simulink model "ExRobotAndEnvironmentController"  (Simulink 8.3)
settings: Solver=ode45  StartTime=0.0  StopTime=1000  FixedStep=.01  RelTol=1e-3
undefined symbols (not defined in the file): Env, INITIAL_ROBOT_POS_THETA, INITIAL_ROBOT_POS_X, INITIAL_ROBOT_POS_Y, INTER_WHEEL_DISTANCE, ki_teta, kp_teta, MAX_SPEED, Robot, RobotInit, ts, ts_anim
libraries: simulink x4
settings Model: Creator=alex  LastModifiedBy=schuhm
settings OptimizationCC: ExpressionDepthLimit=2147483647
settings DebuggingCC: SolverPrmCheckMsg=none  FcnCallInpInsideContextMsg=UseLocalSettings
settings SFSimCC: SimParseCustomCode=off

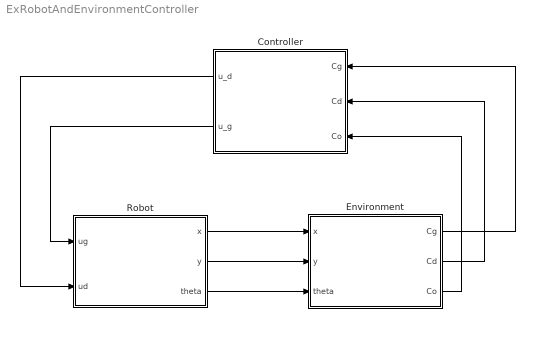
== system ExRobotAndEnvironmentController ==
  Controller : Subsystem
  Environment : Subsystem
  Robot : Subsystem
  wires:
  Robot/1(x) -> Environment/1(x)
  Robot/2(y) -> Environment/2(y)
  Robot/3(theta) -> Environment/3(theta)
  Environment/1(Cg) -> Controller/1(Cg)
  Environment/2(Cd) -> Controller/2(Cd)
  Controller/1(u_d) -> Robot/2(ud)
  Controller/2(u_g) -> Robot/1(ug)
  Environment/3(Co) -> Controller/3(Co)

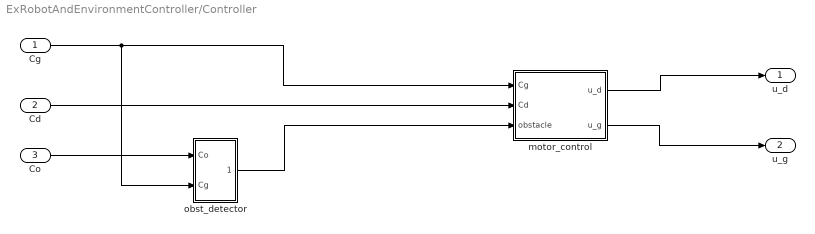
== system ExRobotAndEnvironmentController/Controller ==
  Cg : Inport
  Cd : Inport  Port=2
  Co : Inport  Port=3  OutDataTypeStr=double
  motor_control : Subsystem
  obst_detector : Subsystem
  u_d : Outport
  u_g : Outport  Port=2
  wires:
  Cg/1 -> obst_detector/2(Cg), motor_control/1(Cg)
  Cd/1 -> motor_control/2(Cd)
  obst_detector/1(obstacle) -> motor_control/3(obstacle)
  motor_control/1(u_d) -> u_d/1
  Co/1 -> obst_detector/1(Co)
  motor_control/2(u_g) -> u_g/1

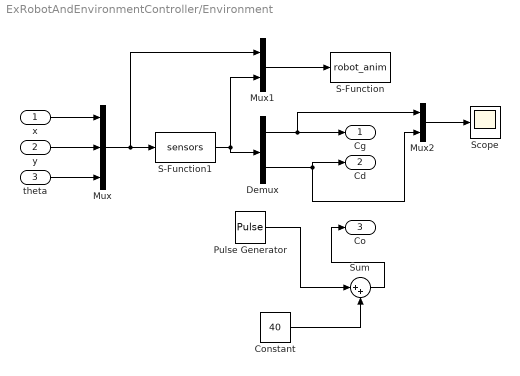
== system ExRobotAndEnvironmentController/Environment ==
  x : Inport
  y : Inport  Port=2
  theta : Inport  Port=3
  Constant : Constant  Value=40
  Demux : Demux  Outputs=2
  Mux : Mux  Inputs=3
  Mux1 : Mux  Inputs=2
  Mux2 : Mux  Inputs=2
  Pulse Generator : DiscretePulseGenerator  PulseType=Time based  Amplitude=-30  Period=5  PulseWidth=5  PhaseDelay=5
  S-Function : S-Function  FunctionName=robot_anim  Parameters=ts_anim,Env,Robot,RobotInit  EnableBusSupport=off
  S-Function1 : S-Function  FunctionName=sensors  Parameters=ts,Env,Robot  EnableBusSupport=off
  Scope : Scope
      settings: TimeRange=25  YMin=0  YMax=100
  Sum : Sum  Inputs=|++
  Cg : Outport
  Cd : Outport  Port=2
  Co : Outport  Port=3
  wires:
  x/1 -> Mux/1
  y/1 -> Mux/2
  theta/1 -> Mux/3
  Mux/1 -> S-Function1/1, Mux1/1
  S-Function1/1 -> Mux1/2, Demux/1
  Mux1/1 -> S-Function/1
  Demux/1 -> Mux2/1, Cg/1
  Demux/2 -> Mux2/2, Cd/1
  Sum/1 -> Co/1
  Pulse Generator/1 -> Sum/1
  Constant/1 -> Sum/2
  Mux2/1 -> Scope/1

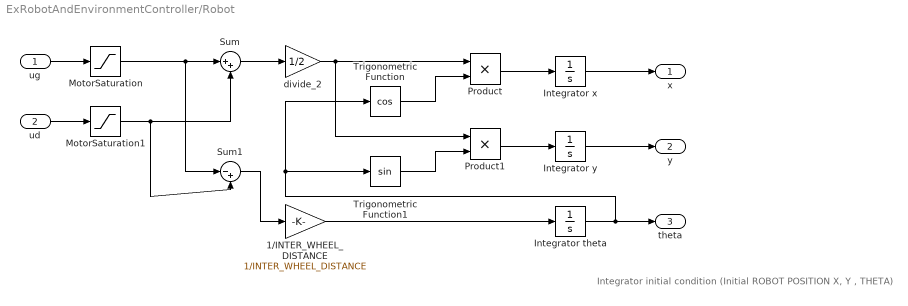
== system ExRobotAndEnvironmentController/Robot ==
  note: Integrator initial condition (Initial ROBOT POSITION X, Y , THETA)
  ug : Inport
  ud : Inport  Port=2
  1/INTER_WHEEL_DISTANCE : Gain  Gain=1/INTER_WHEEL_DISTANCE
  Integrator theta : Integrator  InitialCondition=INITIAL_ROBOT_POS_THETA
  Integrator x : Integrator  InitialCondition=INITIAL_ROBOT_POS_X
  Integrator y : Integrator  InitialCondition=INITIAL_ROBOT_POS_Y
  MotorSaturation : Saturate  UpperLimit=MAX_SPEED  LowerLimit=-MAX_SPEED
  MotorSaturation1 : Saturate  UpperLimit=MAX_SPEED  LowerLimit=-MAX_SPEED
  Product : Product  RndMeth=Zero
  Product1 : Product  RndMeth=Zero
  Sum : Sum  Inputs=|++
  Sum1 : Sum  Inputs=|-+
  Trigonometric Function : Trigonometry  Operator=cos
  Trigonometric Function1 : Trigonometry
  divide_2 : Gain  Gain=1/2
  x : Outport
  y : Outport  Port=2
  theta : Outport  Port=3
  wires:
  ug/1 -> MotorSaturation/1
  Integrator x/1 -> x/1
  Integrator y/1 -> y/1
  Integrator theta/1 -> Trigonometric Function/1, Trigonometric Function1/1, theta/1
  Sum/1 -> divide_2/1
  divide_2/1 -> Product1/1, Product/1
  Trigonometric Function/1 -> Product/2
  Trigonometric Function1/1 -> Product1/2
  Product/1 -> Integrator x/1
  Product1/1 -> Integrator y/1
  Sum1/1 -> 1/INTER_WHEEL_DISTANCE/1
  1/INTER_WHEEL_DISTANCE/1 -> Integrator theta/1
  ud/1 -> MotorSaturation1/1
  MotorSaturation1/1 -> Sum/2, Sum1/2
  MotorSaturation/1 -> Sum/1, Sum1/1

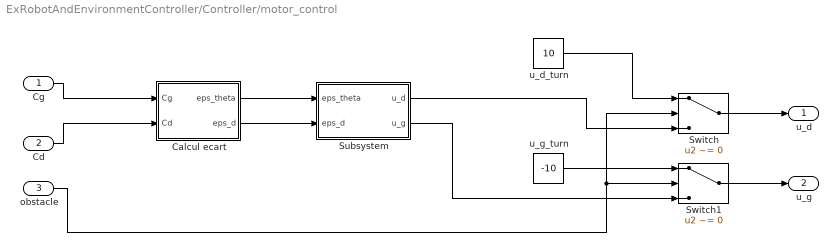
== system ExRobotAndEnvironmentController/Controller/motor_control ==
  Cg : Inport
  Cd : Inport  Port=2
  obstacle : Inport  Port=3
  Calcul ecart : Subsystem
  Subsystem : Subsystem
  Switch : Switch  Criteria=u2 ~= 0
  Switch1 : Switch  Criteria=u2 ~= 0
  u_d_turn : Constant  Value=10
  u_g_turn : Constant  Value=-10
  u_d : Outport
  u_g : Outport  Port=2
  wires:
  obstacle/1 -> Switch/2, Switch1/2
  Calcul ecart/2(eps_d) -> Subsystem/2(eps_d)
  Cd/1 -> Calcul ecart/2(Cd)
  Calcul ecart/1(eps_theta) -> Subsystem/1(eps_theta)
  Cg/1 -> Calcul ecart/1(Cg)
  Subsystem/1(u_d) -> Switch/3
  Switch/1 -> u_d/1
  Subsystem/2(u_g) -> Switch1/3
  Switch1/1 -> u_g/1
  u_g_turn/1 -> Switch1/1
  u_d_turn/1 -> Switch/1

== system ExRobotAndEnvironmentController/Controller/obst_detector ==
  Co : Inport
  Cg : Inport  Port=2
  Obstacle detector : Subsystem
  Unit Delay : UnitDelay  SampleTime=-1
  WBW : Subsystem
  obstacle : Outport
  wires:
  WBW/1(WBW) -> Unit Delay/1
  Unit Delay/1 -> WBW/2(R), Obstacle detector/2(R)
  Co/1 -> Obstacle detector/1(Co)
  Obstacle detector/1(obstacle_detected) -> obstacle/1
  Cg/1 -> WBW/1(Cg)

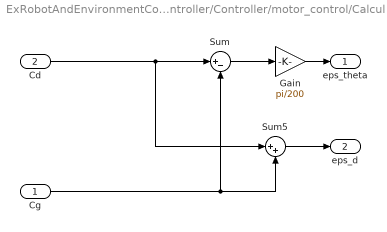
== system ExRobotAndEnvironmentController/Controller/motor_control/Calcul ecart ==
  Cg : Inport
  Cd : Inport  Port=2
  Gain : Gain  Gain=pi/200
  Sum : Sum  Inputs=|+-
  Sum5 : Sum  Inputs=|++
  eps_theta : Outport
  eps_d : Outport  Port=2
  wires:
  Sum/1 -> Gain/1
  Cd/1 -> Sum/1, Sum5/1
  Cg/1 -> Sum/2, Sum5/2
  Gain/1 -> eps_theta/1
  Sum5/1 -> eps_d/1

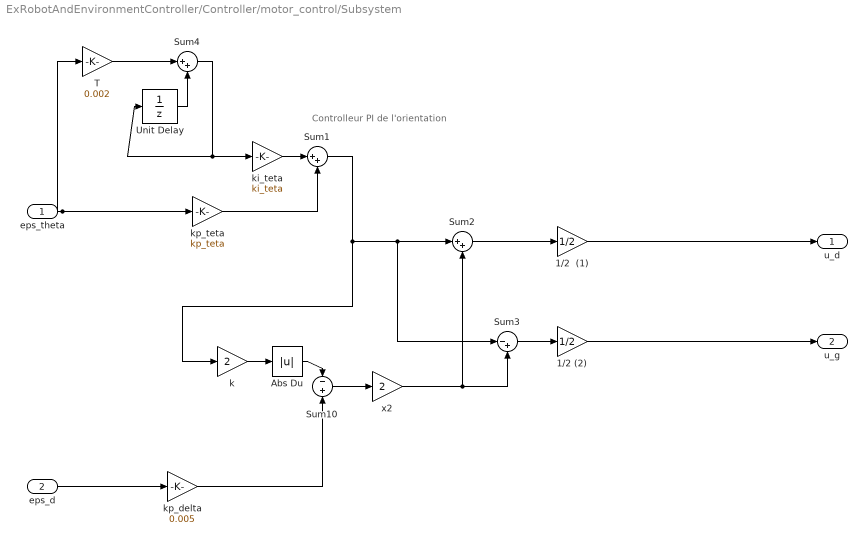
== system ExRobotAndEnvironmentController/Controller/motor_control/Subsystem ==
  note: Controlleur PI de l'orientation
  eps_theta : Inport
  eps_d : Inport  Port=2
  1/2  (1) : Gain  Gain=1/2  SaturateOnIntegerOverflow=on  OutDataTypeStr=Inherit: Same as input  ParamDataTypeStr=Inherit: Same as input
  1/2 (2) : Gain  Gain=1/2  SaturateOnIntegerOverflow=on  OutDataTypeStr=Inherit: Same as input  ParamDataTypeStr=Inherit: Same as input
  Abs Du : Abs  SaturateOnIntegerOverflow=on
  Sum1 : Sum  Inputs=|++  SaturateOnIntegerOverflow=on
  Sum10 : Sum  Inputs=-+  SaturateOnIntegerOverflow=on
  Sum2 : Sum  Inputs=|++  SaturateOnIntegerOverflow=on
  Sum3 : Sum  Inputs=|-+  SaturateOnIntegerOverflow=on
  Sum4 : Sum  Inputs=|++
  T : Gain  Gain=0.002
  Unit Delay : UnitDelay  SampleTime=-1
  k : Gain  Gain=2  SaturateOnIntegerOverflow=on  OutDataTypeStr=Inherit: Same as input  ParamDataTypeStr=Inherit: Same as input
  ki_teta : Gain  Gain=ki_teta  SaturateOnIntegerOverflow=on  OutDataTypeStr=Inherit: Same as input  ParamDataTypeStr=Inherit: Same as input
  kp_delta : Gain  Gain=0.005
  kp_teta : Gain  Gain=kp_teta  SaturateOnIntegerOverflow=on  OutDataTypeStr=Inherit: Same as input  ParamDataTypeStr=Inherit: Same as input
  x2 : Gain  Gain=2  SaturateOnIntegerOverflow=on  OutDataTypeStr=Inherit: Same as input  ParamDataTypeStr=Inherit: Same as input
  u_d : Outport
  u_g : Outport  Port=2
  wires:
  ki_teta/1 -> Sum1/1
  kp_teta/1 -> Sum1/2
  Sum2/1 -> 1/2  (1)/1
  Sum3/1 -> 1/2 (2)/1
  k/1 -> Abs Du/1
  kp_delta/1 -> Sum10/2
  eps_theta/1 -> kp_teta/1, T/1
  Abs Du/1 -> Sum10/1
  x2/1 -> Sum2/2, Sum3/2
  Sum10/1 -> x2/1
  Sum1/1 -> k/1, Sum2/1, Sum3/1
  T/1 -> Sum4/1
  Sum4/1 -> ki_teta/1, Unit Delay/1
  Unit Delay/1 -> Sum4/2
  1/2  (1)/1 -> u_d/1
  1/2 (2)/1 -> u_g/1
  eps_d/1 -> kp_delta/1

== system ExRobotAndEnvironmentController/Controller/obst_detector/Obstacle detector ==
  Co : Inport
  R : Inport  Port=2
  Compare To Constant : simulink/Logic and Bit Operations/Compare To Constant  relop=<  const=20  OutDataTypeStr=boolean
  mem : Subsystem
  obstacle_detected : Outport
  wires:
  Co/1 -> Compare To Constant/1
  mem/1(Q) -> obstacle_detected/1
  R/1 -> mem/2(R)
  Compare To Constant/1 -> mem/1(S)

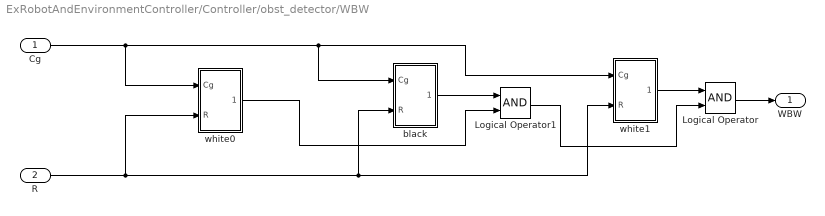
== system ExRobotAndEnvironmentController/Controller/obst_detector/WBW ==
  Cg : Inport
  R : Inport  Port=2
  Logical Operator : Logic  AllPortsSameDT=off  OutDataTypeStr=boolean
  Logical Operator1 : Logic  AllPortsSameDT=off  OutDataTypeStr=boolean
  black : Subsystem
  white0 : Subsystem
  white1 : Subsystem
  WBW : Outport
  wires:
  Cg/1 -> white0/1(Cg), black/1(Cg), white1/1(Cg)
  R/1 -> white0/2(R), white1/2(R), black/2(R)
  black/1(Out1) -> Logical Operator1/1
  white0/1(Out1) -> Logical Operator1/2
  Logical Operator1/1 -> Logical Operator/2
  white1/1(Out1) -> Logical Operator/1
  Logical Operator/1 -> WBW/1

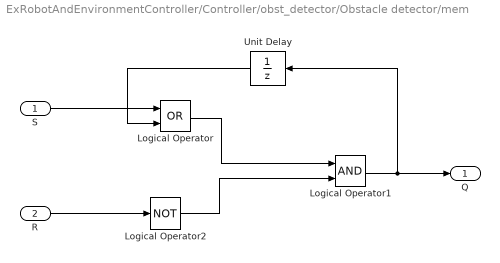
== system ExRobotAndEnvironmentController/Controller/obst_detector/Obstacle detector/mem ==
  S : Inport
  R : Inport  Port=2
  Logical Operator : Logic  Operator=OR  AllPortsSameDT=off  OutDataTypeStr=boolean
  Logical Operator1 : Logic  AllPortsSameDT=off  OutDataTypeStr=boolean
  Logical Operator2 : Logic  Operator=NOT  AllPortsSameDT=off  OutDataTypeStr=boolean
  Unit Delay : UnitDelay  SampleTime=-1
  Q : Outport
  wires:
  Logical Operator/1 -> Logical Operator1/1
  Unit Delay/1 -> Logical Operator/2
  S/1 -> Logical Operator/1
  Logical Operator1/1 -> Q/1, Unit Delay/1
  R/1 -> Logical Operator2/1
  Logical Operator2/1 -> Logical Operator1/2

== system ExRobotAndEnvironmentController/Controller/obst_detector/WBW/black ==
  Cg : Inport
  R : Inport  Port=2
  Compare To Constant : simulink/Logic and Bit Operations/Compare To Constant  relop=<=  const=10  OutDataTypeStr=boolean
  mem : Subsystem
  Out1 : Outport
  wires:
  mem/1(Q) -> Out1/1
  R/1 -> mem/2(R)
  Cg/1 -> Compare To Constant/1
  Compare To Constant/1 -> mem/1(S)

== system ExRobotAndEnvironmentController/Controller/obst_detector/WBW/white0 ==
  Cg : Inport
  R : Inport  Port=2
  Compare To Constant : simulink/Logic and Bit Operations/Compare To Constant  relop=>=  const=90  OutDataTypeStr=boolean
  mem : Subsystem
  Out1 : Outport
  wires:
  mem/1(Q) -> Out1/1
  R/1 -> mem/2(R)
  Cg/1 -> Compare To Constant/1
  Compare To Constant/1 -> mem/1(S)

== system ExRobotAndEnvironmentController/Controller/obst_detector/WBW/white1 ==
  Cg : Inport
  R : Inport  Port=2
  Compare To Constant : simulink/Logic and Bit Operations/Compare To Constant  relop=>=  const=90  OutDataTypeStr=boolean
  mem : Subsystem
  Out1 : Outport
  wires:
  mem/1(Q) -> Out1/1
  R/1 -> mem/2(R)
  Cg/1 -> Compare To Constant/1
  Compare To Constant/1 -> mem/1(S)

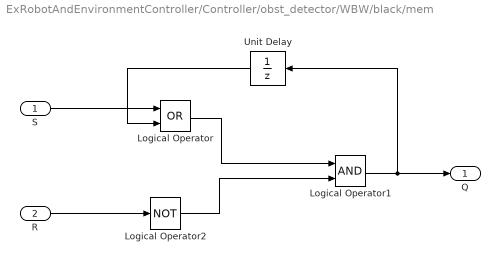
== system ExRobotAndEnvironmentController/Controller/obst_detector/WBW/black/mem ==
  S : Inport
  R : Inport  Port=2
  Logical Operator : Logic  Operator=OR  AllPortsSameDT=off  OutDataTypeStr=boolean
  Logical Operator1 : Logic  AllPortsSameDT=off  OutDataTypeStr=boolean
  Logical Operator2 : Logic  Operator=NOT  AllPortsSameDT=off  OutDataTypeStr=boolean
  Unit Delay : UnitDelay  SampleTime=-1
  Q : Outport
  wires:
  Logical Operator/1 -> Logical Operator1/1
  Unit Delay/1 -> Logical Operator/2
  S/1 -> Logical Operator/1
  Logical Operator1/1 -> Q/1, Unit Delay/1
  R/1 -> Logical Operator2/1
  Logical Operator2/1 -> Logical Operator1/2

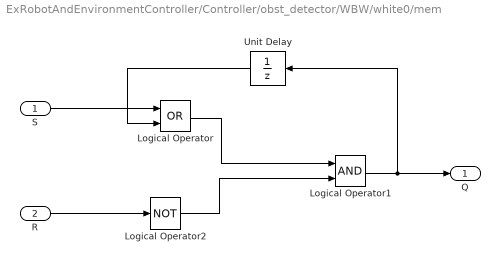
== system ExRobotAndEnvironmentController/Controller/obst_detector/WBW/white0/mem ==
  S : Inport
  R : Inport  Port=2
  Logical Operator : Logic  Operator=OR  AllPortsSameDT=off  OutDataTypeStr=boolean
  Logical Operator1 : Logic  AllPortsSameDT=off  OutDataTypeStr=boolean
  Logical Operator2 : Logic  Operator=NOT  AllPortsSameDT=off  OutDataTypeStr=boolean
  Unit Delay : UnitDelay  SampleTime=-1
  Q : Outport
  wires:
  Logical Operator/1 -> Logical Operator1/1
  Unit Delay/1 -> Logical Operator/2
  S/1 -> Logical Operator/1
  Logical Operator1/1 -> Q/1, Unit Delay/1
  R/1 -> Logical Operator2/1
  Logical Operator2/1 -> Logical Operator1/2

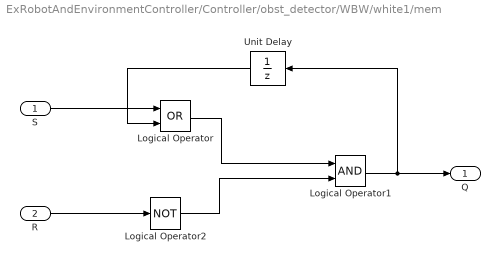
== system ExRobotAndEnvironmentController/Controller/obst_detector/WBW/white1/mem ==
  S : Inport
  R : Inport  Port=2
  Logical Operator : Logic  Operator=OR  AllPortsSameDT=off  OutDataTypeStr=boolean
  Logical Operator1 : Logic  AllPortsSameDT=off  OutDataTypeStr=boolean
  Logical Operator2 : Logic  Operator=NOT  AllPortsSameDT=off  OutDataTypeStr=boolean
  Unit Delay : UnitDelay  SampleTime=-1
  Q : Outport
  wires:
  Logical Operator/1 -> Logical Operator1/1
  Unit Delay/1 -> Logical Operator/2
  S/1 -> Logical Operator/1
  Logical Operator1/1 -> Q/1, Unit Delay/1
  R/1 -> Logical Operator2/1
  Logical Operator2/1 -> Logical Operator1/2
